simulink model "mazeRunner_fixed"  (R2023a)
settings: Solver=FixedStepDiscrete  StartTime=0.0  StopTime=60  FixedStep=0.01  RelTol=1e-3
values from neighbouring files (symbols this model uses):
  axleLength = 0.136    [robotParameters.m]
  maxV = (160/30)*pi*wheelR    (= 0.519409985394)    [robotParameters.m]
  ticksPerRot = 20    [robotParameters.m]
  wheelR = 0.031    [robotParameters.m]
undefined symbols (not defined in the file or in its folder): InputPWM, WheelSpeed
libraries: mobileRoboticsTrainingLib x10, slpidlib x2, simulink x1
settings Model: PacingRate=1000  Creator=friso  LastModifiedBy=friso

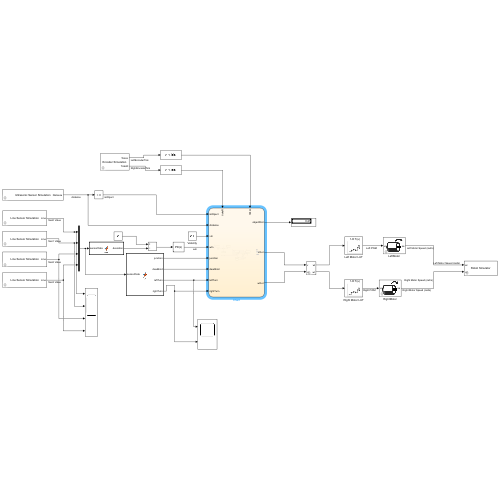
[thumbnail: Simulink's stored preview of the top-level diagram]
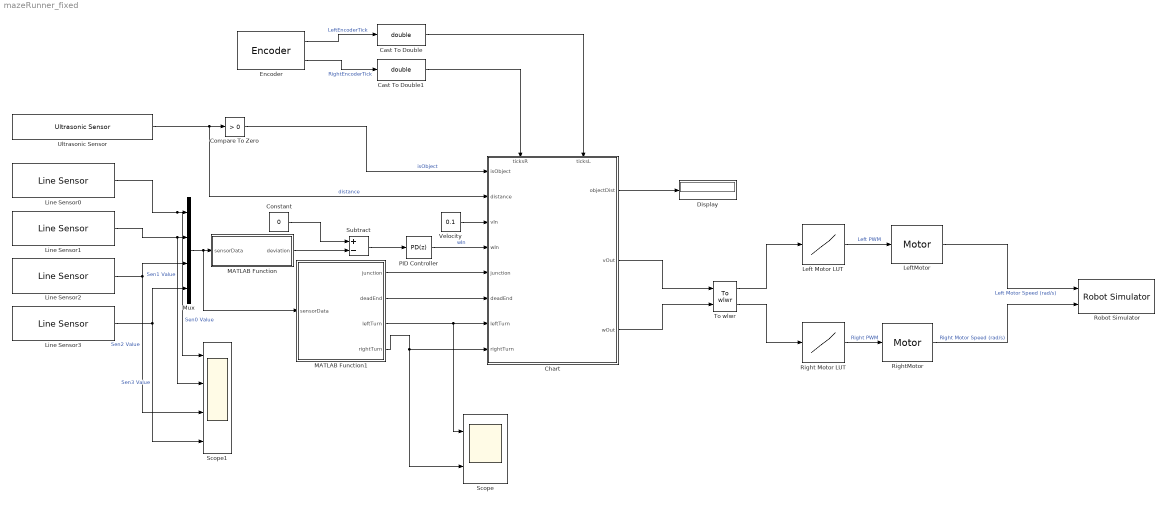
== system mazeRunner_fixed ==
  Cast To Double : DataTypeConversion  OutDataTypeStr=double  SaturateOnIntegerOverflow=off  RndMeth=Floor
  Cast To Double1 : DataTypeConversion  OutDataTypeStr=double  SaturateOnIntegerOverflow=off  RndMeth=Floor
  Chart : Stateflow chart  TreatAsAtomicUnit=on
      settings: PortSchema="{\"entries\":[{\"content\":{\"sides\":[{\"content\":{\"connectorIds\":[\"In3\",\"In2\",\"In9\",\"In10\",\"In4\",\"In1\",\"In5\",\"In6\"]},\"type\":\"ConnectorPlacement.EquallySpacedRectSide\",\"uuid\":\"efd22f5c-d242-47ac-9ce5-ae35ef3018bc\"},{\"content\":{\"connectorIds\":[\"Out1\",\"Out3\",\"Out2\"],\"side\":\"RIGHT\"},\"type\":\"ConnectorPlacement.EquallySpacedRectSide\",\"uuid\":\"ec38a75a-6eb1-4d24-9035-1110e38d6749\"},{\"content\":{\"connectorIds\":[\"In8\",\"In7\"],\"side\":\"TOP\"},\"type\":\"ConnectorPlacement.EquallySpacedRectSide\",\"uuid\":\"4f5603e4-7933-40ac-836c-5b6ac0c06f0e\"},{\"content\":{\"side\":\"BOTTOM\"},\"type\":\"ConnectorPlacement.EquallySpacedRectSide\",\"uuid\":\"3d386817-a5cc-4a0f-aae1-dce75ee13d1b\"}]},\"type\":\"ConnectorPlacement.EquallySpacedConnector\",\"uuid\":\"84912c5f-ccd1-4bed-ad56-74df58d63384\"}],\"packageUris\":[\"http://schema.mathworks.com/mf0/Connector/R2020b\"],\"version\":\"1.0\"}"
  Compare To Zero : simulink/Logic and Bit Operations/Compare To Zero  relop=>  OutDataTypeStr=boolean
  Constant : Constant  Value=0
  Display : Display
  Encoder : mobileRoboticsTrainingLib/Encoder  Priority=2  axleLength=axleLength  wheelR=wheelR  ticksPerRot=ticksPerRot
      settings: SourceProductName=Mobile Robotics Training Library
  Left Motor LUT : Lookup_n-D  NumberOfTableDimensions=1  BreakpointsForDimension1=WheelSpeed  Table=InputPWM  InterpMethod=Nearest  ExtrapMethod=Clip  InternalRulePriority=Speed  RndMeth=Simplest
  LeftMotor : mobileRoboticsTrainingLib/Motor  motorPlant=wheelMotorModel  sensorType=Speed
      settings: SourceProductName=Mobile Robotics Training Library
  Line Sensor0 : mobileRoboticsTrainingLib/Line Sensor  mapVariable=mapForSim  envVal=enviroVal  lineVal=lineVal  sensOff=[0.0643 0.0354]
      settings: SourceProductName=Mobile Robotics Training Library
  Line Sensor1 : mobileRoboticsTrainingLib/Line Sensor  mapVariable=mapForSim  envVal=enviroVal  lineVal=lineVal  sensOff=[0.0675 0.005]
      settings: SourceProductName=Mobile Robotics Training Library
  Line Sensor2 : mobileRoboticsTrainingLib/Line Sensor  mapVariable=mapForSim  envVal=enviroVal  lineVal=lineVal  sensOff=[0.0675 -0.005]
      settings: SourceProductName=Mobile Robotics Training Library
  Line Sensor3 : mobileRoboticsTrainingLib/Line Sensor  mapVariable=mapForSim  envVal=enviroVal  lineVal=lineVal  sensOff=[0.0643 -0.0354]
      settings: SourceProductName=Mobile Robotics Training Library
  MATLAB Function : MATLAB Function  TreatAsAtomicUnit=on
  MATLAB Function1 : MATLAB Function  TreatAsAtomicUnit=on
  Mux : Mux
  PID Controller : slpidlib/PID Controller  Controller=PD  Form=Parallel  TimeDomain=Discrete-time  UseExternalTs=off  SampleTime=-1  IntegratorMethod=Forward Euler  FilterMethod=Forward Euler  ControllerParametersSource=internal  P=10  I=1  UseKiTs=off  D=10e-5  N=100  UseFilter=on  TunerSelectOption=Frequency Response Based  InitialConditionSource=internal  InitialConditionForIntegrator=0  InitialConditionForFilter=0  DifferentiatorICPrevScaledInput=0  ExternalReset=none  TrackingMode=off  Kt=1  LimitOutput=off  SatLimitsSource=internal  UpperSaturationLimit=inf  LowerSaturationLimit=-inf  LinearizeAsGain=on  AntiWindupMode=none  Kb=1  LimitIntegrator=off  UpperIntegratorSaturationLimit=inf  LowerIntegratorSaturationLimit=-inf  POutMin=[]  POutMax=[]  IOutMin=[]  IOutMax=[]  DOutMin=[]  DOutMax=[]  NOutMin=[]  NOutMax=[]  SumOutMin=[]  SumOutMax=[]  SaturationOutMin=[]  SaturationOutMax=[]  PParamMin=[]  PParamMax=[]  IParamMin=[]  IParamMax=[]  DParamMin=[]  DParamMax=[]  NParamMin=[]  NParamMax=[]  KbParamMin=[]  KbParamMax=[]  KtParamMin=[]  KtParamMax=[]  KbOutMin=[]  KbOutMax=[]  KtOutMin=[]  KtOutMax=[]  IntegratorOutMin=[]  IntegratorOutMax=[]  FilterOutMin=[]  FilterOutMax=[]  SumI1OutMin=[]  SumI1OutMax=[]  SumI2OutMin=[]  SumI2OutMax=[]  SumI3OutMin=[]  SumI3OutMax=[]  SumI4OutMin=[]  SumI4OutMax=[]  SumDOutMin=[]  SumDOutMax=[]  DifferentiatorOutMin=[]  DifferentiatorOutMax=[]  FilterDiffOutCoefMin=[]  FilterDiffOutCoefMax=[]  ReciprocalOutMin=[]  ReciprocalOutMax=[]  SumDenOutMin=[]  SumDenOutMax=[]  SumNumOutMin=[]  SumNumOutMax=[]  DivideOutMin=[]  DivideOutMax=[]  UdiffTsProdOutMin=[]  UdiffTsProdOutMax=[]  NTsProdOutMin=[]  NTsProdOutMax=[]  UintegralTsProdOutMin=[]  UintegralTsProdOutMax=[]  UngainTsProdOutMin=[]  UngainTsProdOutMax=[]  ClampingZeroOutDataTypeStr=Inherit: Inherit via back propagation  ClampingZeroOutMin=[]  ClampingZeroOutMax=[]  FilterDenConstantOutDataTypeStr=Inherit: Inherit via back propagation  FilterDenConstantOutMin=[]  FilterDenConstantOutMax=[]  PCopyOutDataTypeStr=Inherit: Inherit via back propagation  PCopyOutMin=[]  PCopyOutMax=[]  NCopyOutDataTypeStr=Inherit: Inherit via back propagation  NCopyOutMin=[]  NCopyOutMax=[]  IntegratorContinuousStateAttributes=''  IntegratorStateMustResolveToSignalObject=off  IntegratorRTWStateStorageClass=Auto  FilterContinuousStateAttributes=''  FilterStateMustResolveToSignalObject=off  FilterRTWStateStorageClass=Auto  ParallelPVariant=InternalParameters  IdealPVariant=Disabled  IVariant=Disabled  DVariant=InternalParameters  IntegratorVariant=Disabled  SatVariant=Disabled  AWVariant=Disabled  PCopyVariant=Disabled  TRVariant=Disabled  FdbkBlocksVariant=Forward  IdealPFdbkVariant=Disabled  SatFdbkVariant=Disabled  DerivativeFilterVariant=ForwardEulerFilter  NVariant=InternalParameters  NCopyVariant=Disabled  FilterICVariant=InternalICsFilter  IntegratorICVariant=Disabled  ExternalResetVariant=Disabled  TRSumVariant=Passthrough  SumFdbkVariant=Disabled  SumVariant=Sum_PD  TsampFilterVariant=InternalTs  TsampNgainVariant=Passthrough  TsampIntegralVariant=Disabled_SignalSpec  ExternalSaturationOutDataTypeStr=Inherit: Same as second input
  Right Motor LUT : Lookup_n-D  NumberOfTableDimensions=1  BreakpointsForDimension1=WheelSpeed  Table=InputPWM  InterpMethod=Nearest  ExtrapMethod=Clip  InternalRulePriority=Speed  RndMeth=Simplest
  RightMotor : mobileRoboticsTrainingLib/Motor  motorPlant=wheelMotorModel  sensorType=Speed
      settings: SourceProductName=Mobile Robotics Training Library
  Robot Simulator : mobileRoboticsTrainingLib/Robot Simulator  Priority=99  mapVar=mapForSim  startX=0.49  startY=0.1  startTheta=90  axleLength=axleLength  wheelR=wheelR
  Scope : Scope  NumInputPorts=2
  Scope1 : Scope  NumInputPorts=4
  Subtract : Sum  Inputs=+-
  To wlwr : mobileRoboticsTrainingLib/To wlwr  axleLength=0.1  wheelR=0.05
  Ultrasonic Sensor : mobileRoboticsTrainingLib/Ultrasonic Sensor  mapVar=mapForSim  maxSenRange=2  minSenRange=0.02  senRes=0.01  sensOff=[0 0]
      settings: SourceProductName=Mobile Robotics Training Library
  Velocity : Constant  Value=0.1
  wires:
  Line Sensor2/1 -> Scope1/3, Mux/3  "Sen2 Value"
  Line Sensor1/1 -> Scope1/2, Mux/2  "Sen1 Value"
  Subtract/1 -> PID Controller/1
  Line Sensor3/1 -> Scope1/4, Mux/4  "Sen3 Value"
  MATLAB Function/1(deviation) -> Subtract/2
  Line Sensor0/1 -> Scope1/1, Mux/1  "Sen0 Value"
  Constant/1 -> Subtract/1
  Mux/1 -> MATLAB Function1/1(sensorData), MATLAB Function/1(sensorData)
  Encoder/1 -> Cast To Double/1  "LeftEncoderTick"
  Encoder/2 -> Cast To Double1/1  "RightEncoderTick"
  Ultrasonic Sensor/1 -> Compare To Zero/1, Chart/2(distance)  "distance"
  Compare To Zero/1 -> Chart/3(isObject)  "isObject"
  PID Controller/1 -> Chart/10(wIn)  "wIn"
  MATLAB Function1/1(junction) -> Chart/4(junction)
  MATLAB Function1/2(deadEnd) -> Chart/1(deadEnd)
  MATLAB Function1/3(leftTurn) -> Scope/1, Chart/5(leftTurn)
  MATLAB Function1/4(rightTurn) -> Scope/2, Chart/6(rightTurn)
  Velocity/1 -> Chart/9(vIn)
  Cast To Double1/1 -> Chart/8(ticksR)
  Cast To Double/1 -> Chart/7(ticksL)
  Chart/1(objectDist) -> Display/1
  LeftMotor/1 -> Robot Simulator/1  "Left Motor Speed (rad/s)"
  Left Motor LUT/1 -> LeftMotor/1  "Left PWM"
  To wlwr/2 -> Right Motor LUT/1
  RightMotor/1 -> Robot Simulator/2  "Right Motor Speed (rad/s)"
  To wlwr/1 -> Left Motor LUT/1
  Right Motor LUT/1 -> RightMotor/1  "Right PWM"
  Chart/3(vOut) -> To wlwr/1
  Chart/2(wOut) -> To wlwr/2

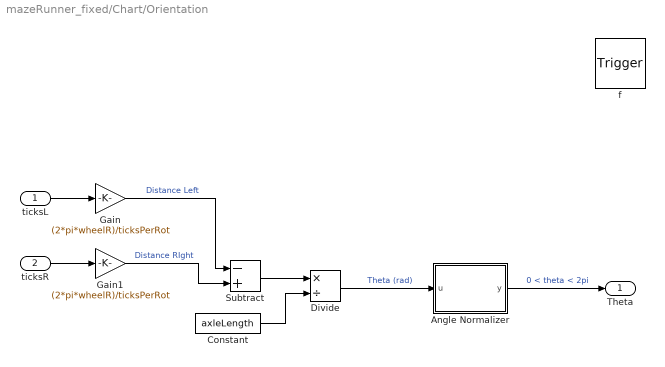
== system mazeRunner_fixed/Chart/Orientation ==
  ticksL : Inport  OutDataTypeStr=double  PortDimensions=1
  ticksR : Inport  Port=2  OutDataTypeStr=double  PortDimensions=1
  f : TriggerPort  TriggerType=function-call  VariantControl=(inherit)
      settings: CopyFcn=Stateflow.SLINSF.SimulinkMan.removeBlockPreDeleteFcn  PreDeleteFcn=Stateflow.SLINSF.SimulinkMan.unsafePredeleteFcn
  Angle Normalizer : MATLAB Function  TreatAsAtomicUnit=on
  Constant : Constant  Value=axleLength
  Divide : Product  Inputs=*/
  Gain : Gain  Gain=(2*pi*wheelR)/ticksPerRot
  Gain1 : Gain  Gain=(2*pi*wheelR)/ticksPerRot
  Subtract : Sum  Inputs=-+
  Theta : Outport
  wires:
  Constant/1 -> Divide/2
  Gain/1 -> Subtract/1  "Distance Left"
  ticksL/1 -> Gain/1
  Angle Normalizer/1(y) -> Theta/1  "0 < theta < 2pi"
  Divide/1 -> Angle Normalizer/1(u)  "Theta (rad)"
  ticksR/1 -> Gain1/1
  Gain1/1 -> Subtract/2  "Distance RIght"
  Subtract/1 -> Divide/1

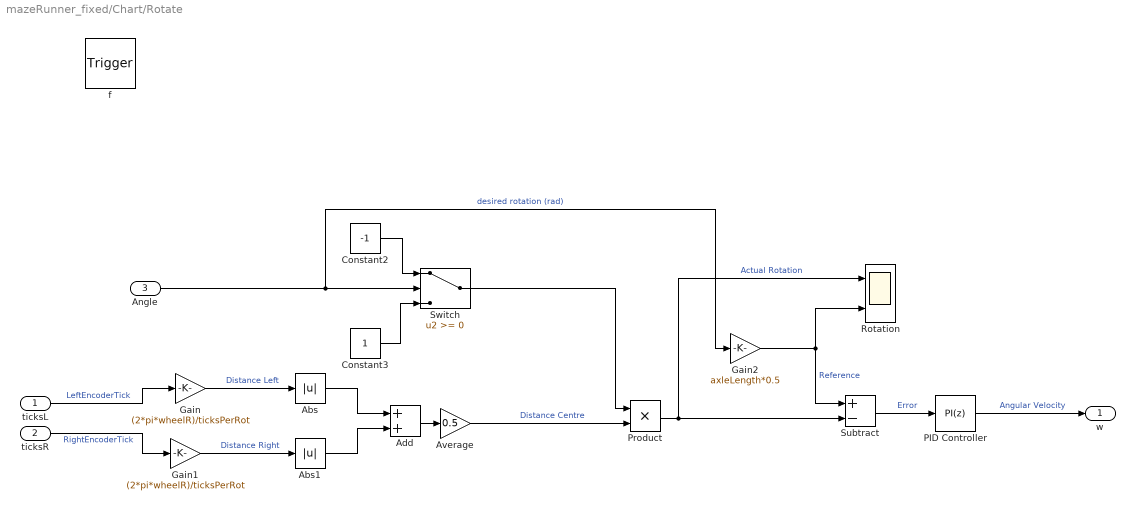
== system mazeRunner_fixed/Chart/Rotate ==
  ticksL : Inport  OutDataTypeStr=double  PortDimensions=1
  ticksR : Inport  Port=2  OutDataTypeStr=double  PortDimensions=1
  Angle : Inport  Port=3  OutDataTypeStr=double  PortDimensions=1
  f : TriggerPort  TriggerType=function-call  VariantControl=(inherit)
      settings: CopyFcn=Stateflow.SLINSF.SimulinkMan.removeBlockPreDeleteFcn  PreDeleteFcn=Stateflow.SLINSF.SimulinkMan.unsafePredeleteFcn
  Abs : Abs  SaturateOnIntegerOverflow=off
  Abs1 : Abs  SaturateOnIntegerOverflow=off
  Add : Sum
  Average : Gain  Gain=0.5
  Constant2 : Constant  Value=-1
  Constant3 : Constant
  Gain : Gain  Gain=(2*pi*wheelR)/ticksPerRot
  Gain1 : Gain  Gain=(2*pi*wheelR)/ticksPerRot
  Gain2 : Gain  Gain=axleLength*0.5
  PID Controller : slpidlib/PID Controller  Controller=PI  Form=Ideal  TimeDomain=Discrete-time  UseExternalTs=off  SampleTime=-1  IntegratorMethod=Forward Euler  FilterMethod=Forward Euler  ControllerParametersSource=internal  P=18  I=0.2  UseKiTs=off  D=0.02  N=100  UseFilter=on  TunerSelectOption=Transfer Function Based (PID Tuner App)  InitialConditionSource=internal  InitialConditionForIntegrator=0  InitialConditionForFilter=0  DifferentiatorICPrevScaledInput=0  ExternalReset=none  TrackingMode=off  Kt=1  LimitOutput=on  SatLimitsSource=internal  UpperSaturationLimit=maxV  LowerSaturationLimit=-maxV  LinearizeAsGain=on  AntiWindupMode=clamping  Kb=1  LimitIntegrator=off  UpperIntegratorSaturationLimit=inf  LowerIntegratorSaturationLimit=-inf  POutMin=[]  POutMax=[]  IOutMin=[]  IOutMax=[]  DOutMin=[]  DOutMax=[]  NOutMin=[]  NOutMax=[]  SumOutMin=[]  SumOutMax=[]  SaturationOutMin=[]  SaturationOutMax=[]  PParamMin=[]  PParamMax=[]  IParamMin=[]  IParamMax=[]  DParamMin=[]  DParamMax=[]  NParamMin=[]  NParamMax=[]  KbParamMin=[]  KbParamMax=[]  KtParamMin=[]  KtParamMax=[]  KbOutMin=[]  KbOutMax=[]  KtOutMin=[]  KtOutMax=[]  IntegratorOutMin=[]  IntegratorOutMax=[]  FilterOutMin=[]  FilterOutMax=[]  SumI1OutMin=[]  SumI1OutMax=[]  SumI2OutMin=[]  SumI2OutMax=[]  SumI3OutMin=[]  SumI3OutMax=[]  SumI4OutMin=[]  SumI4OutMax=[]  SumDOutMin=[]  SumDOutMax=[]  DifferentiatorOutMin=[]  DifferentiatorOutMax=[]  FilterDiffOutCoefMin=[]  FilterDiffOutCoefMax=[]  ReciprocalOutMin=[]  ReciprocalOutMax=[]  SumDenOutMin=[]  SumDenOutMax=[]  SumNumOutMin=[]  SumNumOutMax=[]  DivideOutMin=[]  DivideOutMax=[]  UdiffTsProdOutMin=[]  UdiffTsProdOutMax=[]  NTsProdOutMin=[]  NTsProdOutMax=[]  UintegralTsProdOutMin=[]  UintegralTsProdOutMax=[]  UngainTsProdOutMin=[]  UngainTsProdOutMax=[]  ClampingZeroOutDataTypeStr=Inherit: Inherit via back propagation  ClampingZeroOutMin=[]  ClampingZeroOutMax=[]  FilterDenConstantOutDataTypeStr=Inherit: Inherit via back propagation  FilterDenConstantOutMin=[]  FilterDenConstantOutMax=[]  PCopyOutDataTypeStr=Inherit: Inherit via back propagation  PCopyOutMin=[]  PCopyOutMax=[]  NCopyOutDataTypeStr=Inherit: Inherit via back propagation  NCopyOutMin=[]  NCopyOutMax=[]  IntegratorContinuousStateAttributes=''  IntegratorStateMustResolveToSignalObject=off  IntegratorRTWStateStorageClass=Auto  FilterContinuousStateAttributes=''  FilterStateMustResolveToSignalObject=off  FilterRTWStateStorageClass=Auto  ParallelPVariant=Passthrough  IdealPVariant=InternalParameters  IVariant=InternalParameters  DVariant=Disabled  IntegratorVariant=Discrete  SatVariant=Enabled  AWVariant=DiscClampingIdeal  PCopyVariant=InternalParamsIdeal  TRVariant=Disabled  FdbkBlocksVariant=Forward  IdealPFdbkVariant=Disabled  SatFdbkVariant=Disabled  DerivativeFilterVariant=Disabled  NVariant=Disabled  NCopyVariant=Disabled_SignalSpec  FilterICVariant=Disabled  IntegratorICVariant=InternalICs  ExternalResetVariant=Disabled  TRSumVariant=Passthrough  SumFdbkVariant=Disabled  SumVariant=Sum_PI  TsampFilterVariant=InternalTs  TsampNgainVariant=Passthrough  TsampIntegralVariant=Disabled_SignalSpec  ExternalSaturationOutDataTypeStr=Inherit: Same as second input
  Product : Product
  Rotation : Scope  NumInputPorts=2
  Subtract : Sum  Inputs=+-
  Switch : Switch  Priority=1  SaturateOnIntegerOverflow=off  InputSameDT=off
  w : Outport
  wires:
  Switch/1 -> Product/1
  Add/1 -> Average/1
  ticksR/1 -> Gain1/1  "RightEncoderTick"
  Abs1/1 -> Add/2
  Constant2/1 -> Switch/1
  PID Controller/1 -> w/1  "Angular Velocity"
  Average/1 -> Product/2  "Distance Centre"
  Subtract/1 -> PID Controller/1  "Error"
  Product/1 -> Rotation/1, Subtract/2  "Actual Rotation"
  Angle/1 -> Gain2/1, Switch/2  "desired rotation (rad)"
  Gain/1 -> Abs/1  "Distance Left"
  Abs/1 -> Add/1
  Constant3/1 -> Switch/3
  Gain2/1 -> Subtract/1, Rotation/2  "Reference"
  Gain1/1 -> Abs1/1  "Distance Right"
  ticksL/1 -> Gain/1  "LeftEncoderTick"

== matlab function mazeRunner_fixed/MATLAB Function1 ==
  data: junction output; sensorData input; deadEnd output; leftTurn output; rightTurn output
function [junction, deadEnd, leftTurn, rightTurn]  = fcn(sensorData)
totalZero = 0;
deadEnd = false;
junction = false;
leftTurn = false;
rightTurn = false;

% Change depending on physical sensors
enviroVal = 2800;
lineVal = 2900;

% Total number of Sensors not on line
for i=1:1:size(sensorData, 1)
    if (sensorData(i) == enviroVal)
        totalZero = totalZero + 1;
    end
end

if sensorData(1, 1) == lineVal && sensorData(4, 1) == lineVal
    junction = true; % At junction or detect line (depends on if there is an object or not)
elseif totalZero == size(sensorData, 1) 
    deadEnd = true; % No sensors on line    
end

if sensorData(1,1) == lineVal
    leftTurn = true; % Left high, right low
end
if sensorData(4,1) == lineVal
    rightTurn = true; % Right high, left low
end

% Potentially add count and check if at junction/turn not aligned
% Potentailly add condition for end of maze

== matlab function mazeRunner_fixed/MATLAB Function ==
  data: sensorData input; deviation output
function deviation = fcn(sensorData)
totalZero = 0;
for i=1:1:size(sensorData, 1)
    if (sensorData(i) == 2800)
        totalZero = totalZero + 1;
    end
end

if totalZero == 0
    deviation = -10;
else
    deviation = ((sensorData(1)*-2)+(sensorData(2)*-1)+(sensorData(3)*1)+(sensorData(4)*2))/totalZero;
end

== stateflow chart mazeRunner_fixed/Chart ==
  state turnRight1
    entry:
    thetaInitial = Orientation(ticksL, ticksR); % Angle before rotation
    vOut = 0.02;
    during:
    wOut  = Rotate(ticksL, ticksR, -pi/2);
    rotation = abs(Orientation(ticksL, ticksR) - thetaInitial);
  state turnLeft1
    entry:
    thetaInitial = Orientation(ticksL, ticksR);
    vOut = 0.02;
    during:
    wOut  = Rotate(ticksL, ticksR, pi/2);
    rotation = abs(Orientation(ticksL, ticksR) - abs(thetaInitial));
  state lineFollowing1
    entry, during:
    wOut = wIn  % from PI controller
    vOut = vIn % Constant
    j = 0;
  state atClosestObj
    % various options
    entry:
    wOut = 100;
  state updateCounter
    entry:
    i = i-1;
    during:
    wOut = wIn;
  state turnRight
    entry:
    thetaInitial = Orientation(ticksL, ticksR); % Angle before rotation
    vOut = 0.02;
    during:
    wOut  = Rotate(ticksL, ticksR, -pi/2);
    rotation = abs(Orientation(ticksL, ticksR) - thetaInitial);
  state turnLeft
    entry:
    thetaInitial = Orientation(ticksL, ticksR);
    vOut = 0.02;
    during:
    wOut  = Rotate(ticksL, ticksR, pi/2);
    rotation = abs(Orientation(ticksL, ticksR) - abs(thetaInitial));
  state Theta = Orientation(ticksL,ticksR) [function]
  state turnAround1
    entry:
    thetaInitial = Orientation(ticksL, ticksR); % Angle before rotation
    vOut = 0; % no linear velocity
    during:
    wOut = Rotate(ticksL, ticksR, pi); % Turn 180 degrees
    rotation = abs(Orientation(ticksL, ticksR)- thetaInitial);
  state initialize
    entry:
    thetaInitial = 0;
    objectDist = -1;
    rotation = -1;
    trackerArray = zeros(10, 1);
    i = 1;
    j = 0;
    minDist = 100;
    prevTurn = 1 % 1 = right, -1 = left
    % default: right
  state lineFollowing
    entry, during:
    wOut = wIn  % from PI controller
    vOut = vIn % Constant
    j = 0;
  state atJunction
    % various options
    entry:
    vOut, wOut = 0;
    j = j + 1;
  state w = Rotate(ticksL,ticksR,Angle) [function]
  state finishLine
    entry:
    path = RemoveBranches(trackerArray);
    i = length(path);
  state unoReverse
    entry:
    wOut = 0;
    vOut = -0.03
  state turnAround
    entry:
    thetaInitial = Orientation(ticksL, ticksR); % Angle before rotation
    vOut = 0; % no linear velocity
    during:
    wOut = Rotate(ticksL, ticksR, pi); % Turn 180 degrees
    rotation = abs(Orientation(ticksL, ticksR)- thetaInitial);
  state measureObject
    % Record distance to object
    entry:
    objectDist = distance;
    % Change to be able to hold at least two values
  state Compare
    % Compare distance
    % Clear array
    entry:
    minDist = objectDist;
    trackerArray = zeros(10, 1);
    i = 1;
  (junction 158) -> (junction 154)
  (junction 154) -> (junction 148)
  (junction 152) -> (junction 158)
  turnRight1 -> (junction 152) [order 1] : [leftTurn == true && rotation < pi/12]
  turnLeft1 -> (junction 152) [order 2] : [rightTurn == true && rotation < pi/12]
  turnRight1 -> (junction 150) [order 2]
  turnLeft1 -> (junction 150) [order 1]
  (junction 150) -> lineFollowing1 : [rotation >= pi/2] {rotation = -1; i = i - 1}
  (junction 144) -> turnLeft1 : [leftTurn == true && path(i) == 1]
  (junction 160) -> turnRight1
  lineFollowing1 -> (junction 160) [order 2] : [rightTurn == true && path(i) == -1]
  lineFollowing1 -> (junction 144) [order 1]
  (junction 148) -> atClosestObj
  lineFollowing1 -> updateCounter [order 3] : [rightTurn || leftTurn]
  updateCounter -> lineFollowing1 : after(3.5, sec)
  turnAround1 -> lineFollowing1 : [rotation >= 0.97*pi]{rotation = -1}
  (junction 118) -> (junction 120)
  (junction 116) -> (junction 118)
  (junction 120) -> turnLeft
  (junction 79) -> (junction 83)
  (junction 83) -> (junction 84)
  (junction 76) -> (junction 79)
  turnRight -> (junction 76) [order 1] : [leftTurn == true && rotation < pi/12]
  turnLeft -> (junction 76) [order 2] : [rightTurn == true && rotation < pi/12]
  turnRight -> (junction 64) [order 2] : [rotation >= pi/2]{trackerArray(i, 1) =1 ; prevTurn = 1}
  turnLeft -> (junction 64) [order 1] : [rotation >= pi/2]{trackerArray(i, 1) =-1; prevTurn = -1}
  (junction 64) -> lineFollowing : {rotation = -1; i = i + 1}
  (junction 72) -> turnLeft : [leftTurn == true]
  atJunction -> turnRight [order 3] : [prevTurn == 1]
  (junction 42) -> turnRight
  (default) -> initialize
  finishLine -> turnAround1
  lineFollowing -> (junction 42) [order 4] : [rightTurn == true]
  lineFollowing -> (junction 72) [order 3]
  (junction 84) -> atJunction
  lineFollowing -> atJunction [order 2] : [junction == true]
  initialize -> lineFollowing
  atJunction -> (junction 116) [order 4] : [prevTurn == -1]
  lineFollowing -> unoReverse [order 1] : [deadEnd == true]
  turnAround -> lineFollowing : [rotation >= 0.97*pi]{rotation = -1}
  atJunction -> (junction 135) [order 2]
  atJunction -> measureObject [order 1] : [isObject == true]
  (junction 135) -> finishLine : [j == 50]
  unoReverse -> turnAround : [deadEnd == false]
  measureObject -> turnAround [order 2]
  measureObject -> Compare [order 1] : [objectDist < minDist]
  (junction 112) -> turnAround
  Compare -> (junction 112)
  data: trackerArray function_input; returnPath function_output; ticksL function_input double size=1; ticksR function_input double size=1; Theta function_output; ticksL function_input double size=1; ticksR function_input double size=1; Angle function_input double size=1; w function_output; deadEnd input; distance input; isObject input; junction input; leftTurn input; rightTurn input; ticksL input; ticksR input; vIn input; wIn input; objectDist output size=1; wOut output; thetaInitial local; vOut output; rotation local; i local; trackerArray local; minDist local; prevTurn local; j local; path local size=20 [..20]
  function returnPath = RemoveBranches(trackerArray):
    | function returnPath = RemoveBranches(trackerArray)
    | 
    | returnPath = trackerArray;
    | coder.varsize('returnPath');
    | 
    | for i = length(returnPath):-1:2
    |     if returnPath(i) == 0
    |         returnPath(i) = [];
    |     elseif returnPath(i) == returnPath(i-1)
    |         returnPath(i) = 2;
    |         returnPath(i-1) = [];
    |     end
    | end
    | 
    | end

== matlab function mazeRunner_fixed/Chart/Orientation/Angle Normalizer ==
  data: u input size=1; y output size=1
function y = fcn(u)
if u>2*pi
    y = mod(real(u),2*pi);
else
    y = u;
end
